simulink model "Q3"  (R2025b)
settings: Solver=VariableStepAuto  StartTime=0.0  StopTime=10  RelTol=1e-3
libraries: autolibshared x1
settings Model: Creator=r3anjum  LastModifiedBy=r3anjum

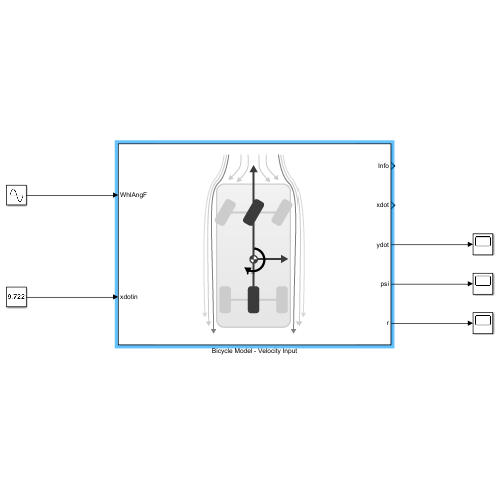
[thumbnail: Simulink's stored preview of the top-level diagram]
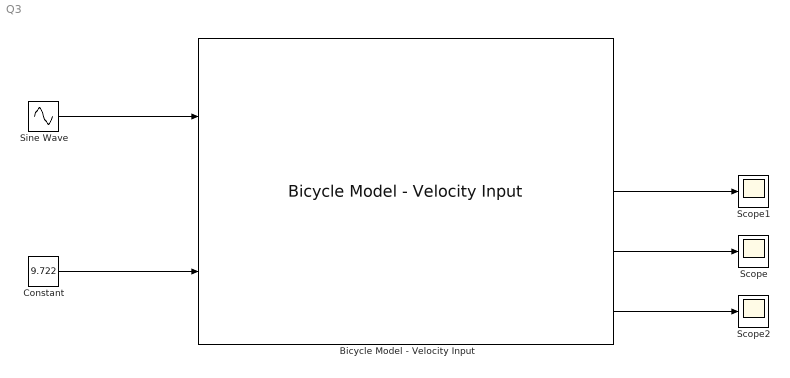
== system Q3 ==
  Bicycle Model - Velocity Input : autolibshared/Bicycle Model - Velocity Input  trackMode=Single (bicycle)  inputMode=External longitudinal velocity  frontSteerMode=on  rearSteerMode=off  windMode=off  muMode=off  extFMode=off  extMMode=off  aMode=2  NF=2  NR=2  m=1590  a=1.18  b=1.77  h=0.72  X_o=0  xdot_o=0  CalphaMode=off  sigmaMode=on  w=[1.4,1.4]  Cy_f=60764.86  Cy_r=41478.59  sigma_f=.1  sigma_r=.1  alpha_f_brk=[-.1 .1]  Cy_f_data=[-9e3 9e3]  alpha_r_brk=[-.1 .1]  Cy_r_data=[-9e3 9e3]  Y_o=0  ydot_o=0  Izz=2687.1  psi_o=0  r_o=0  Af=2  Cd=.3  Cl=.1  Cpm=.1  beta_w=[0 0.01:0.01:0.3]  Cs=[0 0.01:0.01:0.3]  Cym=[0 1e-6:0.01:0.3]  Pabs=101325  Tair=273  g=9.81  mu=1  xdot_tol=.01  Fznom=5000  Fxtire_sat=1e6  Fytire_sat=1e6  longOff=0  latOff=0  vertOff=0
      settings: LibrarySourceBlock=vehdynlibeom/Bicycle Model - Velocity Input
  Constant : Constant  Value=9.722
  Scope : Scope
      settings: ActiveDisplayYMinimum=-0.068946307323235187  ActiveDisplayYMaximum=0.62051676590911686
  Scope1 : Scope
      settings: ActiveDisplayYMinimum=-1  ActiveDisplayYMaximum=1
  Scope2 : Scope
      settings: ActiveDisplayYMinimum=-0.32762893511898128  ActiveDisplayYMaximum=0.32755815970494351  DataLoggingVariableName=ScopeData2
  Sine Wave : Sin  Amplitude=0.06981  Frequency=0.952  SampleTime=0
  wires:
  Sine Wave/1 -> Bicycle Model - Velocity Input/1
  Constant/1 -> Bicycle Model - Velocity Input/2
  Bicycle Model - Velocity Input/4 -> Scope/1
  Bicycle Model - Velocity Input/3 -> Scope1/1
  Bicycle Model - Velocity Input/5 -> Scope2/1
